simulink model "IntegratorSimulink"  (R2018a)
settings: Solver=VariableStepAuto  StartTime=0.0  StopTime=10.0  RelTol=1e-3  EnableMultiTasking=on
values from neighbouring files (symbols this model uses):
  Cair = 0.3    [Data.m]    (also in go.m = 0.4; go_params.m = 0.4)
  dU0 = 0*ones(Usize,1)    [go.m]
  g = 9.8    [Data.m]    (also in go.m; go_params.m)
  M = 288    [Data.m]    (also in go.m; go_params.m)
  Miur0 = 0.01    [Data.m]    (also in go.m; go_params.m)
  pair = 1.25    [Data.m]    (also in go.m = 0.9643; go_params.m = 0.9643)
  Rwr = 0.3302    [Data.m]    (also in go.m = 0.58; go_params.m = 0.58)
  Surf = 0.94243    [Data.m]    (also in go.m; go_params.m)
  U0 = 0*ones(Usize,1)    [go.m]
settings Model: Creator=stajeddi  LastModifiedBy=yesid
settings DataIOCC: LimitDataPoints=on
settings OptimizationCC: LifeSpan=inf
settings DebuggingCC: AllowSymbolicDim=off  SFUnexpectedBacktrackingDiag=warning  SFNoUnconditionalDefaultTransitionDiag=warning  SFExecutionAtInitializationDiag=none
settings ModelReferenceCC: PropagateSignalLabelsOutOfModel=off
settings CodeAppCC: StateflowObjectComments=on
settings GRTTargetCC: TargetLangStandard=C89/C90 (ANSI)
settings ConfigComp: CovMetricSettings=dw  CovHtmlReporting=on  CovSaveCumulativeToWorkspaceVar=on  CovSaveSingleToWorkspaceVar=on  CovExternalEMLEnable=off

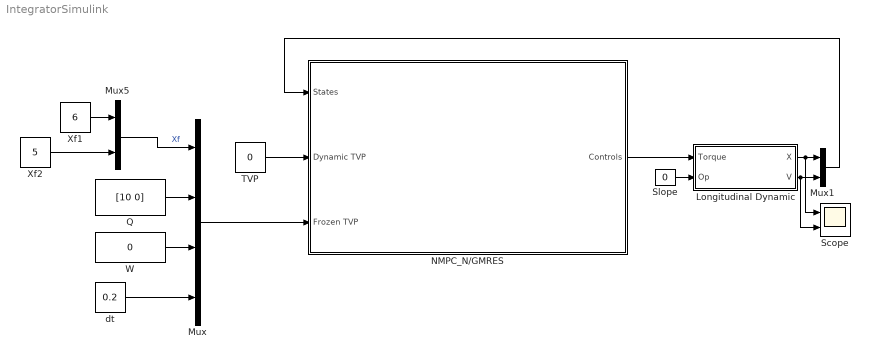
== system IntegratorSimulink ==
  Longitudinal Dynamic : Subsystem
  Mux : Mux
  Mux1 : Mux  Inputs=2
  Mux5 : Mux  Inputs=2
  NMPC_N/GMRES : Subsystem
  Q : Constant  Value=[10 0]
  Scope : Scope  NumInputPorts=2
  Slope : Constant  Value=0
  TVP : Constant  Value=0
  W : Constant  Value=0
  Xf1 : Constant  Value=6
  Xf2 : Constant  Value=5
  dt : Constant  Value=0.2
  wires:
  Mux/1 -> NMPC_N/GMRES/3(Frozen TVP)
  dt/1 -> Mux/4
  Q/1 -> Mux/2
  W/1 -> Mux/3
  Mux5/1 -> Mux/1  "Xf"
  TVP/1 -> NMPC_N/GMRES/2(Dynamic TVP)
  Longitudinal Dynamic/1(X) -> Scope/1, Mux1/1
  NMPC_N/GMRES/1(Controls) -> Longitudinal Dynamic/1(Torque)
  Longitudinal Dynamic/2(V) -> Mux1/2, Scope/2
  Slope/1 -> Longitudinal Dynamic/2("Op ")
  Mux1/1 -> NMPC_N/GMRES/1(States)
  Xf1/1 -> Mux5/1
  Xf2/1 -> Mux5/2

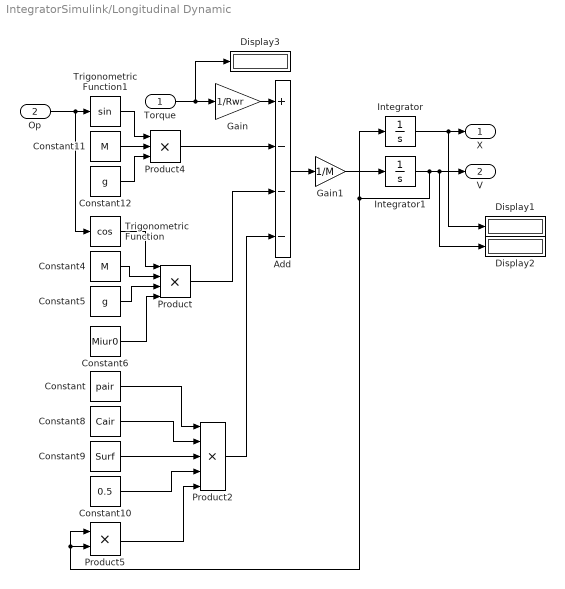
== system IntegratorSimulink/Longitudinal Dynamic ==
  Torque : Inport
  "Op " : Inport  Port=2
  Add : Sum  Inputs=+---
  Constant : Constant  Value=pair
  Constant10 : Constant  Value=0.5
  Constant11 : Constant  Value=M
  Constant12 : Constant  Value=g
  Constant4 : Constant  Value=M
  Constant5 : Constant  Value=g
  Constant6 : Constant  Value=Miur0
  Constant8 : Constant  Value=Cair
  Constant9 : Constant  Value=Surf
  Display1 : Display
  Display2 : Display
  Display3 : Display
  Gain : Gain  Gain=1/Rwr
  Gain1 : Gain  Gain=1/M
  Integrator : Integrator
  Integrator1 : Integrator
  Product : Product  Inputs=4
  Product2 : Product  Inputs=5
  Product4 : Product  Inputs=3
  Product5 : Product
  Trigonometric Function : Trigonometry  Operator=cos
  Trigonometric Function1 : Trigonometry
  X : Outport
  V : Outport  Port=2
  wires:
  Torque/1 -> Display3/1, Gain/1
  Integrator1/1 -> Product5/2, Product5/1, Integrator/1, Display2/1, V/1
  Gain1/1 -> Integrator1/1
  Constant11/1 -> Product4/2
  Trigonometric Function1/1 -> Product4/1
  Constant12/1 -> Product4/3
  Gain/1 -> Add/1
  Product4/1 -> Add/2
  "Op "/1 -> Trigonometric Function/1, Trigonometric Function1/1
  Add/1 -> Gain1/1
  Constant4/1 -> Product/2
  Constant5/1 -> Product/3
  Trigonometric Function/1 -> Product/1
  Constant6/1 -> Product/4
  Product/1 -> Add/3
  Constant9/1 -> Product2/3
  Constant/1 -> Product2/1
  Constant8/1 -> Product2/2
  Constant10/1 -> Product2/4
  Product5/1 -> Product2/5
  Product2/1 -> Add/4
  Integrator/1 -> Display1/1, X/1

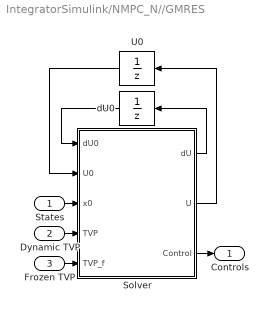
== system IntegratorSimulink/NMPC_N//GMRES ==
  States : Inport
  Dynamic TVP : Inport  Port=2
  Frozen TVP : Inport  Port=3
  Solver : MATLAB Function  TreatAsAtomicUnit=on
  U0 : UnitDelay  InitialCondition=U0  SampleTime=-1
  dU0 : UnitDelay  InitialCondition=dU0  SampleTime=-1
  Controls : Outport
  wires:
  States/1 -> Solver/3(x0)
  Frozen TVP/1 -> Solver/5(TVP_f)
  Solver/3(Control) -> Controls/1
  Solver/2(U) -> U0/1
  U0/1 -> Solver/2(U0)
  Solver/1(dU) -> dU0/1
  dU0/1 -> Solver/1(dU0)
  Dynamic TVP/1 -> Solver/4(TVP)

== matlab function IntegratorSimulink/NMPC_N//GMRES/Solver ==
  data: dU0 input; dU output; U0 input; x0 input; TVP input; U output; Control output; TVP_f input
%% NGMRES  NGMRES NGMRES
function [dU,U,Control] = NMPCBlock(dU0,U0,x0,TVP,TVP_f)
[dU,U,Control]=NMPC(dU0,U0,x0,TVP,TVP_f);
